simulink library "AEMS_Standard_Library"  (R2016b)
settings: Solver=ode45  StartTime=0.0  StopTime=10.0  RelTol=1e-3
undefined symbols (not defined in the file or in its folder): BkPY, carto, Cbx_extegr, Cbx_lpegrsys, Cbx_portegr, Cnx_bnk_nr_conf, Cnx_cyl_nr_conf, ConfigManagement, configuration_management, Cxx_dcm_io_tmr_end_xxxx, Cxx_dcm_rt_tmr_end, Cxx_DID_xxxx_IO_max, Cxx_DID_xxxx_IO_min, Cxx_egrhsofs, Cxx_vmaniegi, DEM_DEBOUNCE_FREEZE, DEM_DTR_CTL_INVISIBLE, DEM_DTR_CTL_NORMAL, Dem_DtrId2_XXX, Dem_DtrId3_XXX, Dem_DtrId4_XXX, Dem_DtrId5_XXX, Dem_DtrId6_XXX, Dem_DtrId7_XXX, Dem_DtrId8_XXX, Dem_DtrId9_XXX, Dem_DtrId_XXX, Dem_EnableConditionId2_XXX, Dem_EnableConditionId3_XXX, Dem_EnableConditionId4_XXX, Dem_EnableConditionId5_XXX, Dem_EnableConditionId6_XXX, Dem_EnableConditionId7_XXX, Dem_EnableConditionId8_XXX, Dem_EnableConditionId_XXX, Dem_EventId, Dem_EventId2_XXX, Dem_EventId3_XXX, Dem_EventId4_XXX, Dem_EventId5_XXX, Dem_EventId6_XXX, Dem_EventId7_XXX, Dem_EventId8_XXX, Dem_EventId9_XXX, Dem_EventId_Device_Faulttype, Dem_EventId_XXX, DEM_IUMPR_GENERAL_DENOMINATOR, DEM_OPCYC_IGNITION, Dem_RatioId2_XXX, Dem_RatioId3_XXX, Dem_RatioId4_XXX, Dem_RatioId5_XXX, Dem_RatioId6_XXX, Dem_RatioId7_XXX, Dem_RatioId8_XXX, Dem_RatioId_XXX, Dem_StorageConditionId2_XXX, Dem_StorageConditionId3_XXX, Dem_StorageConditionId4_XXX, Dem_StorageConditionId5_XXX ... (+65)
libraries: AEMS_Standard_Library x477, simulink x2
(part 17 of 39)

== system AEMS_Standard_Library/FILTER/AEMS_FILTER_WITH_DELAY_CONTROL ==
  filter_param : Inport
  kp : Inport  Port=2
  input : Inport  Port=3
  timestep : Inport  Port=4
  AEMS_SLEW_RATE : AEMS_Standard_Library/DISCONTINUITIES/AEMS_SLEW_RATE  Tag=[LIB]
      settings: AttributesFormatString=%<MaskType>
  Constant1 : Constant  Value=true
  DivisionByZero : Subsystem  Tag=[LIB]
  First_Order_Filter : Subsystem
  First_Order_Filter1 : Subsystem
  First_Order_Filter2 : Subsystem
  LogicalOperator2 : Logic  Operator=NOT  Inputs=1  OutDataTypeStr=boolean
  MinMax1 : MinMax  Function=max  Inputs=2  OutDataTypeStr=Inherit: Inherit via back propagation  RndMeth=Zero  InputSameDT=on
  MinMax2 : MinMax  Inputs=2  OutDataTypeStr=Inherit: Inherit via back propagation  RndMeth=Zero  InputSameDT=on
  Product : Product  OutDataTypeStr=Inherit: Inherit via back propagation  RndMeth=Zero
  Sum : Sum  Inputs=+-  OutDataTypeStr=Inherit: Inherit via back propagation  RndMeth=Zero  InputSameDT=on
  Sum2 : Sum  OutDataTypeStr=Inherit: Inherit via back propagation  RndMeth=Zero  InputSameDT=on
  Sum3 : Sum  Inputs=-+  OutDataTypeStr=Inherit: Inherit via back propagation  RndMeth=Zero  InputSameDT=on
  Sum5 : Sum  OutDataTypeStr=Inherit: Inherit via back propagation  RndMeth=Zero  InputSameDT=on
  UnitDelay : UnitDelay  SampleTime=-1
      settings: AttributesFormatString=IC = %<X0>
  UnitDelay1 : UnitDelay  SampleTime=-1
      settings: AttributesFormatString=IC = %<X0>
  Unit_Delay1 : UnitDelay  InitialCondition=false  SampleTime=-1
      settings: AttributesFormatString=IC = %<X0>
  g2 : Constant  Value=0  OutDataTypeStr=Inherit: Inherit via back propagation
  g4 : Constant  Value=0  OutDataTypeStr=Inherit: Inherit via back propagation
  g6 : Constant  Value=0  OutDataTypeStr=Inherit: Inherit via back propagation
  output : Outport
  wires:
  First_Order_Filter1/1(output) -> First_Order_Filter2/2(input)
  First_Order_Filter/1(output) -> First_Order_Filter1/2(input)
  filter_param/1 -> First_Order_Filter/1(filter_parameter), First_Order_Filter1/1(filter_parameter), First_Order_Filter2/1(filter_parameter)
  LogicalOperator2/1 -> First_Order_Filter/3(initial), First_Order_Filter1/3(initial), First_Order_Filter2/3(initial)
  Unit_Delay1/1 -> LogicalOperator2/1
  Constant1/1 -> Unit_Delay1/1
  First_Order_Filter2/1(output) -> UnitDelay1/1, Sum3/2
  input/1 -> AEMS_SLEW_RATE/2, Sum/1, First_Order_Filter/2(input)
  Sum3/1 -> DivisionByZero/2(num)
  Sum5/1 -> MinMax1/1
  DivisionByZero/1(ans) -> Sum5/1, Sum2/1
  UnitDelay/1 -> Sum/2
  MinMax1/1 -> AEMS_SLEW_RATE/1
  MinMax2/1 -> AEMS_SLEW_RATE/3
  kp/1 -> Product/2
  Sum/1 -> Product/1
  UnitDelay1/1 -> Sum3/1
  g2/1 -> MinMax1/2
  g4/1 -> MinMax2/2
  AEMS_SLEW_RATE/1 -> output/1, UnitDelay/1
  timestep/1 -> AEMS_SLEW_RATE/4, DivisionByZero/3(den)
  Sum2/1 -> MinMax2/1
  Product/1 -> Sum5/2, Sum2/2
  g6/1 -> DivisionByZero/1(ans_of_0div)

== system AEMS_Standard_Library/FILTER/AEMS_FIRST_ORDER_FILTER_RST ==
  Filter_param : Inport
  Input : Inport  Port=2
  IC : Inport  Port=3
  R : Inport  Port=4
  AEMS_UNITDELAY_RESET_EXTERNALIC : AEMS_Standard_Library/DISCRETE/AEMS_UNITDELAY_RESET_EXTERNALIC  Tag=[LIB]
      settings: AttributesFormatString=%<MaskType>
  Constant1 : Constant  Value=true
  Constant2 : Constant  OutDataTypeStr=Inherit: Inherit via back propagation
  LogicalOperator1 : Logic  Operator=OR  OutDataTypeStr=boolean
  LogicalOperator2 : Logic  Operator=NOT  Inputs=1  OutDataTypeStr=boolean
  Product1 : Product  OutDataTypeStr=single  RndMeth=Zero
  Product2 : Product  OutDataTypeStr=single  RndMeth=Zero
  Sum : Sum  Inputs=+-  OutDataTypeStr=single  RndMeth=Zero  InputSameDT=on
  Sum1 : Sum  OutDataTypeStr=single  RndMeth=Zero  InputSameDT=on
  Switch : Switch  Criteria=u2 ~= 0  RndMeth=Zero  SaturateOnIntegerOverflow=on  InputSameDT=on
      settings: AttributesFormatString=Criteria=%<Criteria>
  Unit_Delay1 : UnitDelay  InitialCondition=false  SampleTime=-1
      settings: AttributesFormatString=<initial=%<InitialCondition>>
  Output : Outport
  wires:
  LogicalOperator2/1 -> LogicalOperator1/2
  LogicalOperator1/1 -> Switch/2
  R/1 -> AEMS_UNITDELAY_RESET_EXTERNALIC/2, LogicalOperator1/1
  Switch/1 -> AEMS_UNITDELAY_RESET_EXTERNALIC/1, Output/1
  IC/1 -> AEMS_UNITDELAY_RESET_EXTERNALIC/3, Switch/1
  Sum1/1 -> Switch/3
  Product2/1 -> Sum1/2
  Product1/1 -> Sum1/1
  Unit_Delay1/1 -> LogicalOperator2/1
  Constant1/1 -> Unit_Delay1/1
  Filter_param/1 -> Product2/1, Sum/2
  Constant2/1 -> Sum/1
  Input/1 -> Product2/2
  Sum/1 -> Product1/2
  AEMS_UNITDELAY_RESET_EXTERNALIC/1 -> Product1/1

== system AEMS_Standard_Library/FILTER/AEMS_FORWARD_EULER_INTEGRATOR_WITH_RESET ==
  note: External reset: "level"
  note: Forward Euler: y(n) = x(n-1)*T*K + y(n-1)
  x : Inport
  Reset : Inport  Port=2
  IC : Inport  Port=3
  uppersaturation : Inport  Port=4
  lowersaturation : Inport  Port=5
  Sample_Time : Inport  Port=6
  Gain_K : Inport  Port=7
  AEMS_CLAMP1 : AEMS_Standard_Library/MATH/AEMS_CLAMP  Tag=[LIB]
      settings: AttributesFormatString=%<MaskType>
  AEMS_UNITDELAY_EXTERNALIC : AEMS_Standard_Library/DISCRETE/AEMS_UNITDELAY_EXTERNALIC  Tag=[LIB]
      settings: AttributesFormatString=%<MaskType>
  Add1 : Sum  OutDataTypeStr=Inherit: Inherit via back propagation  RndMeth=Zero  InputSameDT=on
  LogicalOperator1 : Logic  Operator=OR  OutDataTypeStr=boolean
  Product1 : Product  OutDataTypeStr=Inherit: Inherit via back propagation  RndMeth=Zero
  Product2 : Product  OutDataTypeStr=Inherit: Inherit via back propagation  RndMeth=Zero
  Switch1 : Switch  Criteria=u2 ~= 0  RndMeth=Zero  InputSameDT=on
      settings: AttributesFormatString=Criteria=%<Criteria>
  UnitDelay1 : UnitDelay  SampleTime=-1
      settings: AttributesFormatString=IC = %<X0>
  UnitDelay2 : UnitDelay  SampleTime=-1
      settings: AttributesFormatString=IC = %<X0>
  y : Outport
  wires:
  AEMS_UNITDELAY_EXTERNALIC/1 -> Add1/1
  Product2/1 -> Add1/2
  lowersaturation/1 -> AEMS_CLAMP1/3
  uppersaturation/1 -> AEMS_CLAMP1/1
  Reset/1 -> LogicalOperator1/1, UnitDelay1/1
  UnitDelay1/1 -> LogicalOperator1/2
  IC/1 -> Switch1/1, AEMS_UNITDELAY_EXTERNALIC/2
  x/1 -> UnitDelay2/1
  Sample_Time/1 -> Product1/2
  UnitDelay2/1 -> Product1/1
  Product1/1 -> Product2/1
  Gain_K/1 -> Product2/2
  Add1/1 -> Switch1/3
  LogicalOperator1/1 -> Switch1/2
  Switch1/1 -> AEMS_CLAMP1/2
  AEMS_CLAMP1/1 -> AEMS_UNITDELAY_EXTERNALIC/1, y/1

== system AEMS_Standard_Library/FILTER/AEMS_TAU_TO_FILTER_PARAM ==
  note: Nxb_fil_para = [0.0 0.125 0.25 0.375 0.5 0.625 0.75 0.875 1.0]
  note: Nxp_fil_para = [1.0 0.882497 0.7788 0.687289 0.606531 0.535261 0.472366 0.416862 0.367879]
  Tau : Inport
  Timestep : Inport  Port=2
  AEMS_LUT_1D : AEMS_Standard_Library/LOOKUP_TABLES/AEMS_LUT_1D  Tag=[LIB]  map_x=Nxb_fil_para  map_z=Nxp_fil_para
      settings: AttributesFormatString=%<MaskType>\nBkPX=%<map_x>\nLUT=%<map_z>
  Constant1 : Constant  Value=0  OutDataTypeStr=single
  Constant13 : Constant  OutDataTypeStr=single
  Constant2 : Constant  Value=1.1920929e-07  OutDataTypeStr=single
  Constant3 : Constant  OutDataTypeStr=single
  Divide : Product  Inputs=*/  OutDataTypeStr=Inherit: Inherit via back propagation  RndMeth=Zero
  MinMax : MinMax  Function=max  Inputs=2  OutDataTypeStr=Inherit: Inherit via back propagation  RndMeth=Zero  InputSameDT=on
  RelationalOperator : RelationalOperator  Operator=>  OutDataTypeStr=boolean  RndMeth=Nearest  InputSameDT=on
  Saturation : Saturate  UpperLimit=1  LowerLimit=0  RndMeth=Zero
      settings: AttributesFormatString=L_Limit = %<LowerLimit>\nU_Limit = %<UpperLimit>
  Sum1 : Sum  Inputs=+-  OutDataTypeStr=Inherit: Inherit via back propagation  RndMeth=Zero  InputSameDT=on
  Switch : Switch  Criteria=u2 ~= 0  RndMeth=Zero  SaturateOnIntegerOverflow=on  InputSameDT=on
      settings: AttributesFormatString=Criteria=%<Criteria>
  Filter_param : Outport
  wires:
  Sum1/1 -> Switch/1
  RelationalOperator/1 -> Switch/2
  Constant1/1 -> RelationalOperator/2
  Divide/1 -> Saturation/1
  Tau/1 -> MinMax/1, RelationalOperator/1
  Timestep/1 -> Divide/1
  Constant2/1 -> MinMax/2
  MinMax/1 -> Divide/2
  Saturation/1 -> AEMS_LUT_1D/1
  Switch/1 -> Filter_param/1
  Constant13/1 -> Sum1/1
  AEMS_LUT_1D/1 -> Sum1/2
  Constant3/1 -> Switch/3

== system AEMS_Standard_Library/FILTER/AEMS_TAU_TO_FILTER_PARAM_EXP ==
  Tau : Inport
  Timestep : Inport  Port=2
  Constant : Constant  Value=-1  OutDataTypeStr=Inherit: Inherit via back propagation
  Constant1 : Constant  Value=0  OutDataTypeStr=single
  Constant13 : Constant  OutDataTypeStr=single
  Constant2 : Constant  Value=1.1920929e-07  OutDataTypeStr=single
  Constant3 : Constant  OutDataTypeStr=single
  Divide : Product  Inputs=*/  OutDataTypeStr=Inherit: Inherit via back propagation  RndMeth=Zero
  MathFunction : Math  RndMeth=Zero  SaturateOnIntegerOverflow=on
  MinMax : MinMax  Function=max  Inputs=2  OutDataTypeStr=Inherit: Inherit via back propagation  RndMeth=Zero  InputSameDT=on
  Product : Product  OutDataTypeStr=Inherit: Inherit via back propagation  RndMeth=Zero
  RelationalOperator : RelationalOperator  Operator=>  OutDataTypeStr=boolean  RndMeth=Nearest  InputSameDT=on
  Saturation : Saturate  UpperLimit=1  LowerLimit=0  RndMeth=Zero
      settings: AttributesFormatString=L_Limit = %<LowerLimit>\nU_Limit = %<UpperLimit>
  Sum1 : Sum  Inputs=+-  OutDataTypeStr=Inherit: Inherit via back propagation  RndMeth=Zero  InputSameDT=on
  Switch : Switch  Criteria=u2 ~= 0  RndMeth=Zero  SaturateOnIntegerOverflow=on  InputSameDT=on
      settings: AttributesFormatString=Criteria=%<Criteria>
  Filter_param : Outport
  wires:
  Sum1/1 -> Switch/1
  RelationalOperator/1 -> Switch/2
  Constant1/1 -> RelationalOperator/2
  Divide/1 -> Saturation/1
  Tau/1 -> MinMax/1, RelationalOperator/1
  Timestep/1 -> Divide/1
  Constant2/1 -> MinMax/2
  MinMax/1 -> Divide/2
  Product/1 -> MathFunction/1
  Switch/1 -> Filter_param/1
  Constant13/1 -> Sum1/1
  MathFunction/1 -> Sum1/2
  Constant3/1 -> Switch/3
  Saturation/1 -> Product/1
  Constant/1 -> Product/2

== system AEMS_Standard_Library/FLAG/AEMS_SRFLIPFLOP ==
  S : Inport
  R : Inport  Port=2
  LogicalOperator : Logic  Operator=NOR  OutDataTypeStr=boolean
  LogicalOperator1 : Logic  Operator=NOR  OutDataTypeStr=boolean
  UnitDelay1 : UnitDelay  InitialCondition=InitValue  SampleTime=-1
      settings: AttributesFormatString=IC = %<X0>
  Q : Outport  InitialOutput=1
  wires:
  UnitDelay1/1 -> LogicalOperator/1
  S/1 -> LogicalOperator/2
  LogicalOperator/1 -> LogicalOperator1/1
  LogicalOperator1/1 -> Q/1, UnitDelay1/1
  R/1 -> LogicalOperator1/2

== system AEMS_Standard_Library/HYSTERESIS/AEMS_HYST_DELTARIGHT ==
  note: Hysteresis Model
  val : Inport
      settings: AttributesFormatString=<tsample=%<SampleTime>>
  thrs : Inport  Port=2
      settings: AttributesFormatString=<tsample=%<SampleTime>>
  hysw : Inport  Port=3
      settings: AttributesFormatString=<tsample=%<SampleTime>>
  NOT : Logic  Operator=NOT  Inputs=1  OutDataTypeStr=boolean
  Sum : Sum  SaturateOnIntegerOverflow=on
  Switch : Switch  Criteria=u2 ~= 0  SaturateOnIntegerOverflow=on  InputSameDT=on
      settings: AttributesFormatString=Criteria=%<Criteria>
  Unit Delay : UnitDelay  SampleTime=-1
      settings: AttributesFormatString=<initial=%<X0>>
  hflg=OFF : RelationalOperator  Operator=<=  OutDataTypeStr=boolean  RndMeth=Nearest  InputSameDT=on
  hflg=ON : RelationalOperator  Operator=>  OutDataTypeStr=boolean  RndMeth=Nearest  InputSameDT=on
  flg_ret : Outport
  wires:
  Unit Delay/1 -> Switch/2
  hflg=OFF/1 -> Switch/3
  hflg=ON/1 -> Switch/1
  hysw/1 -> Sum/2  "hysw"
  Switch/1 -> NOT/1
  NOT/1 -> Unit Delay/1, flg_ret/1  "flg_ret"
  Sum/1 -> hflg=ON/2
  thrs/1 -> hflg=ON/1, hflg=OFF/2  "thrs"
  val/1 -> Sum/1, hflg=OFF/1  "val"

== system AEMS_Standard_Library/HYSTERESIS/AEMS_HYST_LEFTDELTA ==
  note: Hysteresis Model
  val : Inport
      settings: AttributesFormatString=<tsample=%<SampleTime>>
  thrs : Inport  Port=2
      settings: AttributesFormatString=<tsample=%<SampleTime>>
  hysw : Inport  Port=3
      settings: AttributesFormatString=<tsample=%<SampleTime>>
  NOT : Logic  Operator=NOT  Inputs=1  OutDataTypeStr=boolean
  Sum : Sum  Inputs=+-  SaturateOnIntegerOverflow=on
  Switch : Switch  Criteria=u2 ~= 0  SaturateOnIntegerOverflow=on  InputSameDT=on
      settings: AttributesFormatString=Criteria=%<Criteria>
  Unit Delay : UnitDelay  SampleTime=-1
      settings: AttributesFormatString=<initial=%<X0>>
  hflg=OFF : RelationalOperator  Operator=<  OutDataTypeStr=boolean  RndMeth=Nearest  InputSameDT=on
  hflg=ON : RelationalOperator  OutDataTypeStr=boolean  RndMeth=Nearest  InputSameDT=on
  flg_ret : Outport
  wires:
  Unit Delay/1 -> NOT/1
  NOT/1 -> Switch/2
  hysw/1 -> Sum/2  "hysw"
  Sum/1 -> hflg=OFF/2
  hflg=OFF/1 -> Switch/1
  hflg=ON/1 -> Switch/3
  Switch/1 -> Unit Delay/1, flg_ret/1  "flg_ret"
  val/1 -> Sum/1, hflg=ON/1  "val"
  thrs/1 -> hflg=OFF/1, hflg=ON/2  "thrs"

== system AEMS_Standard_Library/HYSTERESIS/AEMS_HYST_LEFTRIGHT ==
  Input : Inport  Tag=AM,In,0,1,Name,C;CMP,Port,PortWidth,SampleTime;
  Low_Threshold : Inport  Tag=AM,In,0,1,Name,C;CMP,Port,PortWidth,SampleTime;  Port=2
  High_Threshold : Inport  Tag=AM,In,0,1,Name,C;CMP,Port,PortWidth,SampleTime;  Port=3
  Constant1 : Constant  Value=false
  Logical_Operator2 : Logic  Operator=OR  OutDataTypeStr=boolean
  Relational_Operator : RelationalOperator  Tag=AM,Std,2,1;CMP,Operator;  Operator=>  OutDataTypeStr=boolean  RndMeth=Nearest  InputSameDT=on
  Relational_Operator1 : RelationalOperator  Tag=AM,Std,2,1;CMP,Operator;  Operator=>  OutDataTypeStr=boolean  RndMeth=Nearest  InputSameDT=on
  Switch2 : Switch  Tag=GEN,Threshold;AM,Switch,2,1;CMP,Threshold;  Criteria=u2 ~= 0  RndMeth=Zero  SaturateOnIntegerOverflow=on  InputSameDT=on
      settings: AttributesFormatString=Criteria=%<Criteria>
  Unit Delay : UnitDelay  InitialCondition=InitValue  SampleTime=-1
      settings: AttributesFormatString=<initial=%<X0>>
  Output : Outport  Tag=AM,Out,1,0,Name,NC;CMP,Port,OutputWhenDisabled,InitialOutput;
  wires:
  Low_Threshold/1 -> Relational_Operator/1
  High_Threshold/1 -> Relational_Operator1/2
  Input/1 -> Relational_Operator/2, Relational_Operator1/1
  Relational_Operator/1 -> Switch2/2
  Relational_Operator1/1 -> Logical_Operator2/1
  Constant1/1 -> Switch2/1
  Switch2/1 -> Unit Delay/1, Output/1
  Logical_Operator2/1 -> Switch2/3
  Unit Delay/1 -> Logical_Operator2/2

== system AEMS_Standard_Library/LOOKUP_TABLES/AEMS_DIRECTLU_1D ==
  Index_Ratio : Inport
  Table : Inport  Port=2
  Bus Selector : BusSelector  OutputSignals=Index,Ratio
  Interp (1D) Using PreLookUp : Interpolation_n-D  NumberOfTableDimensions=1  TableSource=Input port  Table=LUT  ExtrapMethod=Clip  RemoveProtectionIndex=on  ValidIndexMayReachLast=on  OutDataTypeStr=Inherit: Inherit via back propagation  RndMeth=Zero  SaturateOnIntegerOverflow=on  TableDataTypeStr=Inherit: Inherit from 'Table data'
      settings: AttributesFormatString=Interpolation method : %<InterpMethod>\nExtrapolation method : %<ExtrapMethod>\nRounding mode : %<RndMeth>  InputPortMap=u0,u1,p2
  Value : Outport
  wires:
  Table/1 -> Interp (1D) Using PreLookUp/3
  Index_Ratio/1 -> Bus Selector/1
  Bus Selector/2 -> Interp (1D) Using PreLookUp/2  "<Ratio>"
  Bus Selector/1 -> Interp (1D) Using PreLookUp/1  "<Index>"
  Interp (1D) Using PreLookUp/1 -> Value/1

== system AEMS_Standard_Library/LOOKUP_TABLES/AEMS_DIRECTLU_2D ==
  Index_Ratio_X : Inport
  Index_Ratio_Y : Inport  Port=2
  MAP : Inport  Port=3
  Bus Selector X : BusSelector  OutputSignals=Index,Ratio
  Bus Selector Y : BusSelector  OutputSignals=Index,Ratio
  Interp (2D) Using PreLookUp : Interpolation_n-D  TableSource=Input port  Table=LUT  ExtrapMethod=Clip  RemoveProtectionIndex=on  ValidIndexMayReachLast=on  OutDataTypeStr=Inherit: Inherit via back propagation  RndMeth=Zero  SaturateOnIntegerOverflow=on  TableDataTypeStr=Inherit: Inherit from 'Table data'
      settings: AttributesFormatString=Interpolation method : %<InterpMethod>\nExtrapolation method : %<ExtrapMethod>\nRounding mode : %<RndMeth>  InputPortMap=u0,u1,u2,u3,p2
  Value : Outport
  wires:
  Index_Ratio_X/1 -> Bus Selector X/1
  Index_Ratio_Y/1 -> Bus Selector Y/1
  Interp (2D) Using PreLookUp/1 -> Value/1
  Bus Selector X/1 -> Interp (2D) Using PreLookUp/1  "<Index>"
  Bus Selector X/2 -> Interp (2D) Using PreLookUp/2  "<Ratio>"
  Bus Selector Y/1 -> Interp (2D) Using PreLookUp/3  "<Index>"
  Bus Selector Y/2 -> Interp (2D) Using PreLookUp/4  "<Ratio>"
  MAP/1 -> Interp (2D) Using PreLookUp/5

== system AEMS_Standard_Library/LOOKUP_TABLES/AEMS_DIRECTLU_INDEXED_1D ==
  Index_Ratio : Inport
  Table : Inport  Port=2
  Bus Selector : BusSelector  OutputSignals=Index
  Direct Look-Up Table (1D) : LookupNDDirect  NumberOfTableDimensions=1  TableIsInput=on  Table=LUT  DiagnosticForOutOfRangeInput=None
      settings: LockScale=on
  Value : Outport
  wires:
  Direct Look-Up Table (1D)/1 -> Value/1
  Bus Selector/1 -> Direct Look-Up Table (1D)/1  "<Index>"
  Index_Ratio/1 -> Bus Selector/1
  Table/1 -> Direct Look-Up Table (1D)/2

== system AEMS_Standard_Library/LOOKUP_TABLES/AEMS_DIRECTLU_INDEXED_2D ==
  Index_Ratio_X : Inport
  Index_Ratio_Y : Inport  Port=2
  MAP : Inport  Port=3
  Bus Selector X : BusSelector  OutputSignals=Index
  Bus Selector Y : BusSelector  OutputSignals=Index
  Direct Look-Up Table (2D) : LookupNDDirect  TableIsInput=on  Table=LUT  DiagnosticForOutOfRangeInput=None
      settings: LockScale=on
  Value : Outport
  wires:
  Index_Ratio_X/1 -> Bus Selector X/1
  Index_Ratio_Y/1 -> Bus Selector Y/1
  Direct Look-Up Table (2D)/1 -> Value/1
  Bus Selector X/1 -> Direct Look-Up Table (2D)/1  "<Index>"
  Bus Selector Y/1 -> Direct Look-Up Table (2D)/2  "<Index>"
  MAP/1 -> Direct Look-Up Table (2D)/3

== system AEMS_Standard_Library/LOOKUP_TABLES/AEMS_DYNAMIC_LUT_1D ==
  Var : Inport
  BkPX : Inport  Port=2
  LUT : Inport  Port=3
  LookupTableDynamic : simulink/Lookup Tables/Lookup Table Dynamic  LookUpMeth=Interpolation-Use End Values  OutDataType=fixdt('double')  OutScaling=[]  OutDataTypeStr=Inherit: Inherit via back propagation  DoSatur=off
      settings: AttributesFormatString=LU Method : %<LookUpMeth>\nRounding mode : %<RndMeth>
  Interp1D : Outport
  wires:
  LookupTableDynamic/1 -> Interp1D/1
  Var/1 -> LookupTableDynamic/1
  BkPX/1 -> LookupTableDynamic/2
  LUT/1 -> LookupTableDynamic/3

== system AEMS_Standard_Library/LOOKUP_TABLES/AEMS_INDEXED_LUT_1D ==
  Var : Inport
  LookupTableIndexed1D : Lookup_n-D  NumberOfTableDimensions=1  BreakpointsForDimension1=map_x  BreakpointsForDimension2=BkPY  BreakpointsForDimension1DataTypeStr=Inherit: Inherit from 'Breakpoint data'  BreakpointsForDimension2DataTypeStr=Inherit: Inherit from 'Breakpoint data'  Table=map_z  TableDataTypeStr=Inherit: Inherit from 'Table data'  InterpMethod=Flat  ExtrapMethod=Clip  UseLastTableValue=on  OutDataTypeStr=Inherit: Inherit via back propagation  RndMeth=Zero  SaturateOnIntegerOverflow=on
      settings: AttributesFormatString="Interpolation method : %<interpMethod>\\nExtrapolation method : %<extrapMethod>\\nBkPX = %<bp1>\\nMAP  = %<tableData>"
  Index1D : Outport
  wires:
  Var/1 -> LookupTableIndexed1D/1
  LookupTableIndexed1D/1 -> Index1D/1

== system AEMS_Standard_Library/LOOKUP_TABLES/AEMS_INDEXED_LUT_1D_TOL ==
  Var : Inport
  AEMS_SRFLIPFLOP : AEMS_Standard_Library/FLAG/AEMS_SRFLIPFLOP  Tag=[LIB]  init=true
      settings: AttributesFormatString=|
      | %<MaskType>
      | Initial condition (state of Q): %<init>
  Constant6 : Constant
  Logical Operator1 : Logic  OutDataTypeStr=boolean
  Lookup Table Indexed (1D) : Lookup_n-D  NumberOfTableDimensions=1  BreakpointsForDimension1=map_x  BreakpointsForDimension2=BkPY  BreakpointsForDimension1DataTypeStr=Inherit: Inherit from 'Breakpoint data'  BreakpointsForDimension2DataTypeStr=Inherit: Inherit from 'Breakpoint data'  Table=map_z  TableDataTypeStr=Inherit: Inherit from 'Table data'  InterpMethod=Flat  ExtrapMethod=Clip  UseLastTableValue=on  OutDataTypeStr=Inherit: Inherit via back propagation  RndMeth=Zero  SaturateOnIntegerOverflow=on
      settings: AttributesFormatString="Interpolation method : %<interpMethod>\\nExtrapolation method : %<extrapMethod>\\nBkPX = %<bp1>\\nMAP  = %<tableData>"
  PreLookUpX : Subsystem
  PreLookUpX+Tol : Subsystem
  Relational Operator1 : RelationalOperator  Operator=~=  OutDataTypeStr=boolean  RndMeth=Nearest  InputSameDT=on
  Relational Operator3 : RelationalOperator  Operator===  OutDataTypeStr=boolean  RndMeth=Nearest  InputSameDT=on
  Relational Operator5 : RelationalOperator  Operator===  OutDataTypeStr=boolean  RndMeth=Nearest  InputSameDT=on
  Sum2 : Sum  SaturateOnIntegerOverflow=on
  Sum6 : Sum  Inputs=+-  RndMeth=Zero  SaturateOnIntegerOverflow=on
  Switch : Switch  Criteria=u2 ~= 0  SaturateOnIntegerOverflow=on
      settings: AttributesFormatString=Criteria=%<Criteria>
  Unit Delay1 : UnitDelay  SampleTime=-1
  Unit Delay2 : UnitDelay  SampleTime=-1
  X_Tolerance : Constant  Value=Tolerance
  Result : Outport
  wires:
  X_Tolerance/1 -> Sum2/1
  PreLookUpX+Tol/1(k) -> Relational Operator3/1
  Lookup Table Indexed (1D)/1 -> Result/1
  Switch/1 -> Lookup Table Indexed (1D)/1
  Relational Operator3/1 -> Unit Delay2/1, Relational Operator1/1, AEMS_SRFLIPFLOP/2
  AEMS_SRFLIPFLOP/1 -> Switch/2
  Unit Delay2/1 -> Relational Operator1/2
  Relational Operator1/1 -> Logical Operator1/2
  Relational Operator5/1 -> Logical Operator1/1
  Logical Operator1/1 -> AEMS_SRFLIPFLOP/1
  Var/1 -> PreLookUpX/1(u), Switch/3, Sum2/2
  Sum2/1 -> PreLookUpX+Tol/1(u), Switch/1
  Sum6/1 -> Relational Operator5/1
  Constant6/1 -> Relational Operator5/2
  Unit Delay1/1 -> Sum6/1
  PreLookUpX/1(k) -> Sum6/2, Unit Delay1/1, Relational Operator3/2

== system AEMS_Standard_Library/LOOKUP_TABLES/AEMS_INDEXED_LUT_2D ==
  VarX : Inport
  VarY : Inport  Port=2
  Lookup Table Indexed (2D) : Lookup_n-D  BreakpointsForDimension1=map_x  BreakpointsForDimension2=map_y  BreakpointsForDimension1DataTypeStr=Inherit: Inherit from 'Breakpoint data'  BreakpointsForDimension2DataTypeStr=Inherit: Inherit from 'Breakpoint data'  Table=carto  TableDataTypeStr=Inherit: Inherit from 'Table data'  InterpMethod=Flat  ExtrapMethod=Clip  UseLastTableValue=on  OutDataTypeStr=Inherit: Inherit via back propagation  RndMeth=Zero  SaturateOnIntegerOverflow=on
      settings: AttributesFormatString="Interpolation method : %<interpMethod>\\nExtrapolation Method : %<extrapMethod>\\nBkPX = %<bp1>\\nBkPY =  %<bp2>\\nMAP  = %<tableData>"
  Index2D : Outport
  wires:
  Lookup Table Indexed (2D)/1 -> Index2D/1
  VarX/1 -> Lookup Table Indexed (2D)/1
  VarY/1 -> Lookup Table Indexed (2D)/2

== system AEMS_Standard_Library/LOOKUP_TABLES/AEMS_INDEXED_LUT_2D_TOL ==
  VarX : Inport
  VarY : Inport  Port=2
  AEMS_SRFLIPFLOPIC : AEMS_Standard_Library/FLAG/AEMS_SRFLIPFLOP  Tag=[LIB]  init=true
      settings: AttributesFormatString=|
      | %<MaskType>
      | Initial condition (state of Q): %<init>
  AEMS_SRFLIPFLOPIC1 : AEMS_Standard_Library/FLAG/AEMS_SRFLIPFLOP  Tag=[LIB]  init=true
      settings: AttributesFormatString=|
      | %<MaskType>
      | Initial condition (state of Q): %<init>
  Constant1 : Constant
  Constant6 : Constant
  Logical Operator1 : Logic  AllPortsSameDT=off
  Logical Operator2 : Logic  AllPortsSameDT=off
  Lookup Table Indexed (2D) : Lookup_n-D  BreakpointsForDimension1=map_x  BreakpointsForDimension2=map_y  BreakpointsForDimension1DataTypeStr=Inherit: Inherit from 'Breakpoint data'  BreakpointsForDimension2DataTypeStr=Inherit: Inherit from 'Breakpoint data'  Table=carto  TableDataTypeStr=Inherit: Inherit from 'Table data'  InterpMethod=Flat  ExtrapMethod=Clip  UseLastTableValue=on  OutDataTypeStr=Inherit: Inherit via back propagation  RndMeth=Zero  SaturateOnIntegerOverflow=on
      settings: AttributesFormatString="Interpolation method : %<interpMethod>\\nExtrapolation Method : %<extrapMethod>\\nBkPX = %<bp1>\\nBkPY =  %<bp2>\\nMAP  = %<tableData>"
  PreLookUpX : Subsystem
  PreLookUpX+Tol : Subsystem
  PreLookUpY : Subsystem
  PreLookUpY+Tol1 : Subsystem
  Relational Operator1 : RelationalOperator  Operator=~=  OutDataTypeStr=boolean  RndMeth=Nearest
  Relational Operator2 : RelationalOperator  Operator=~=  OutDataTypeStr=boolean  RndMeth=Nearest
  Relational Operator{3..6} (4 alike) : RelationalOperator  Operator===  OutDataTypeStr=boolean  RndMeth=Nearest
  Sum1 : Sum  SaturateOnIntegerOverflow=on
  Sum2 : Sum  SaturateOnIntegerOverflow=on
  Sum3 : Sum  Inputs=+-  RndMeth=Zero  SaturateOnIntegerOverflow=on
  Sum6 : Sum  Inputs=+-  RndMeth=Zero  SaturateOnIntegerOverflow=on
  Switch1 : Switch  Threshold=0.5  SaturateOnIntegerOverflow=on
      settings: AttributesFormatString=<threshold=%<threshold>>\n
  Switch2 : Switch  Threshold=0.5  SaturateOnIntegerOverflow=on
      settings: AttributesFormatString=<threshold=%<threshold>>\n
  Unit Delay{1..4} (4 alike) : UnitDelay  SampleTime=-1
  X_Tolerance : Constant  Tag=AM,Constant,0,1,Value;CMP,Value;  Value=X_Tolerance
  Y_Tolerance2 : Constant  Tag=AM,Constant,0,1,Value;CMP,Value;  Value=Y_Tolerance
  Result : Outport
  wires:
  Y_Tolerance2/1 -> Sum1/1
  PreLookUpY+Tol1/1(k) -> Relational Operator4/1
  Relational Operator4/1 -> AEMS_SRFLIPFLOPIC1/2, Unit Delay4/1, Relational Operator2/1
  AEMS_SRFLIPFLOPIC1/1 -> Switch1/2
  Unit Delay4/1 -> Relational Operator2/2
  Relational Operator2/1 -> Logical Operator2/2
  Relational Operator6/1 -> Logical Operator2/1
  Logical Operator2/1 -> AEMS_SRFLIPFLOPIC1/1
  VarY/1 -> Switch1/3, Sum1/2, PreLookUpY/1(u)
  Sum1/1 -> Switch1/1, PreLookUpY+Tol1/1(u)
  Sum3/1 -> Relational Operator6/1
  Constant1/1 -> Relational Operator6/2
  Unit Delay3/1 -> Sum3/1
  PreLookUpY/1(k) -> Sum3/2, Unit Delay3/1, Relational Operator4/2
  X_Tolerance/1 -> Sum2/1
  PreLookUpX+Tol/1(k) -> Relational Operator3/1
  Lookup Table Indexed (2D)/1 -> Result/1
  Switch1/1 -> Lookup Table Indexed (2D)/2
  Switch2/1 -> Lookup Table Indexed (2D)/1
  Relational Operator3/1 -> AEMS_SRFLIPFLOPIC/2, Unit Delay2/1, Relational Operator1/1
  AEMS_SRFLIPFLOPIC/1 -> Switch2/2
  Unit Delay2/1 -> Relational Operator1/2
  Relational Operator1/1 -> Logical Operator1/2
  Relational Operator5/1 -> Logical Operator1/1
  Logical Operator1/1 -> AEMS_SRFLIPFLOPIC/1
  VarX/1 -> PreLookUpX/1(u), Switch2/3, Sum2/2
  Sum2/1 -> PreLookUpX+Tol/1(u), Switch2/1
  Sum6/1 -> Relational Operator5/1
  Constant6/1 -> Relational Operator5/2
  Unit Delay1/1 -> Sum6/1
  PreLookUpX/1(k) -> Sum6/2, Unit Delay1/1, Relational Operator3/2

== system AEMS_Standard_Library/LOOKUP_TABLES/AEMS_INTERP ==
  input_of_ratio_1 : Inport
      settings: AttributesFormatString=<tsample=%<sampleTime>>
  interpolate_ratio : Inport  Port=2
      settings: AttributesFormatString=<tsample=%<sampleTime>>
  input_of_ratio_0 : Inport  Port=3
      settings: AttributesFormatString=<tsample=%<sampleTime>>
  Constant1 : Constant  OutDataTypeStr=Inherit: Inherit via back propagation
  Product : Product  SaturateOnIntegerOverflow=on  RndMeth=Zero  InputSameDT=on
  Product1 : Product  SaturateOnIntegerOverflow=on  RndMeth=Zero  InputSameDT=on
  Saturation : Saturate  UpperLimit=1  LowerLimit=0
      settings: AttributesFormatString=<limits=%<UpperLimit>/%<LowerLimit>>
  Sum : Sum  Inputs=-+  SaturateOnIntegerOverflow=on  InputSameDT=on
  Sum1 : Sum  SaturateOnIntegerOverflow=on  InputSameDT=on
  output : Outport
  wires:
  Sum1/1 -> output/1  "output"
  Constant1/1 -> Sum/2
  input_of_ratio_0/1 -> Product1/2  "input_of_ratio_0"
  Product1/1 -> Sum1/2
  Product/1 -> Sum1/1
  Sum/1 -> Product1/1
  interpolate_ratio/1 -> Saturation/1  "interpolate_ratio"
  input_of_ratio_1/1 -> Product/1  "input_of_ratio_1"
  Saturation/1 -> Product/2, Sum/1  "limited_interpolate_ratio"

== system AEMS_Standard_Library/LOOKUP_TABLES/AEMS_ITP3D ==
  Vxx_fac : Inport
  Vxx_in1 : Inport  Port=2
  Vxx_in2 : Inport  Port=3
  Vxx_in3 : Inport  Port=4
  DataTypeConversion : DataTypeConversion  OutDataTypeStr=uint8  SaturateOnIntegerOverflow=on  RndMeth=Zero
  DataTypeConversion2 : DataTypeConversion  OutDataTypeStr=uint8  SaturateOnIntegerOverflow=on  RndMeth=Zero
  MultiportSwitch : MultiPortSwitch  RndMeth=Zero  SaturateOnIntegerOverflow=on  InputSameDT=on
      settings: AttributesFormatString=PortOrder=%<DataPortOrder>
  MultiportSwitch1 : MultiPortSwitch  RndMeth=Zero  SaturateOnIntegerOverflow=on  InputSameDT=on
      settings: AttributesFormatString=PortOrder=%<DataPortOrder>
  Product : Product  OutDataTypeStr=Inherit: Inherit via back propagation  RndMeth=Zero
  RoundingFunction : Rounding
      settings: AttributesFormatString=Function = %<Operator>
  RoundingFunction1 : Rounding  Operator=ceil
      settings: AttributesFormatString=Function = %<Operator>
  Saturation : Saturate  UpperLimit=3  LowerLimit=1  RndMeth=Zero
      settings: AttributesFormatString=L_Limit = %<LowerLimit>\nU_Limit = %<UpperLimit>
  Sum : Sum  Inputs=+-  OutDataTypeStr=Inherit: Inherit via back propagation  RndMeth=Zero  InputSameDT=on
  Sum1 : Sum  Inputs=+-  OutDataTypeStr=Inherit: Inherit via back propagation  RndMeth=Zero  InputSameDT=on
  Sum2 : Sum  OutDataTypeStr=Inherit: Inherit via back propagation  RndMeth=Zero  InputSameDT=on
  Vxx_out : Outport
  wires:
  DataTypeConversion2/1 -> MultiportSwitch/1
  DataTypeConversion/1 -> MultiportSwitch1/1
  MultiportSwitch/1 -> Sum2/2, Sum1/2
  RoundingFunction/1 -> DataTypeConversion2/1, Sum/2
  RoundingFunction1/1 -> DataTypeConversion/1
  Vxx_in2/1 -> MultiportSwitch1/3, MultiportSwitch/3
  Vxx_in3/1 -> MultiportSwitch1/4, MultiportSwitch/4
  Sum1/1 -> Product/2
  MultiportSwitch1/1 -> Sum1/1
  Vxx_in1/1 -> MultiportSwitch1/2, MultiportSwitch/2
  Sum2/1 -> Vxx_out/1
  Product/1 -> Sum2/1
  Sum/1 -> Product/1
  Saturation/1 -> Sum/1, RoundingFunction/1, RoundingFunction1/1
  Vxx_fac/1 -> Saturation/1

== system AEMS_Standard_Library/LOOKUP_TABLES/AEMS_LUT_1D ==
  Var : Inport
  LookupTable1D : Lookup_n-D  NumberOfTableDimensions=1  BreakpointsForDimension1=map_x  BreakpointsForDimension2=BkPY  BreakpointsForDimension1DataTypeStr=Inherit: Inherit from 'Breakpoint data'  BreakpointsForDimension2DataTypeStr=Inherit: Inherit from 'Breakpoint data'  Table=map_z  TableDataTypeStr=Inherit: Inherit from 'Table data'  ExtrapMethod=Clip  UseLastTableValue=on  OutDataTypeStr=Inherit: Inherit via back propagation  RndMeth=Zero  SaturateOnIntegerOverflow=on
      settings: AttributesFormatString="Interpolation method : %<interpMethod>\\nExtrapolation method : %<extrapMethod>\\nBkPX = %<bp1>\\nMAP  = %<tableData>"
  Interp1D : Outport
  wires:
  Var/1 -> LookupTable1D/1
  LookupTable1D/1 -> Interp1D/1

== system AEMS_Standard_Library/LOOKUP_TABLES/AEMS_LUT_2D ==
  VarX : Inport
  VarY : Inport  Port=2
  Lookup Table (2D) : Lookup_n-D  BreakpointsForDimension1=map_x  BreakpointsForDimension2=map_y  BreakpointsForDimension1DataTypeStr=Inherit: Inherit from 'Breakpoint data'  BreakpointsForDimension2DataTypeStr=Inherit: Inherit from 'Breakpoint data'  Table=carto  TableDataTypeStr=Inherit: Inherit from 'Table data'  ExtrapMethod=Clip  UseLastTableValue=on  OutDataTypeStr=Inherit: Inherit via back propagation  RndMeth=Zero  SaturateOnIntegerOverflow=on
      settings: AttributesFormatString="LU method : %<interpMethod>\\nExtrapolation Method : %<extrapMethod>\\nBkPX = %<bp1>\\nBkPY =  %<bp2>\\nMAP  = %<tableData>"
  Interp2D : Outport
  wires:
  Lookup Table (2D)/1 -> Interp2D/1
  VarX/1 -> Lookup Table (2D)/1
  VarY/1 -> Lookup Table (2D)/2

== system AEMS_Standard_Library/LOOKUP_TABLES/AEMS_PRE_INTERP ==
  Var : Inport
  Bus Creator : BusCreator  Inputs=2  NonVirtualBus=on
      settings: AttributesFormatString=%<OutDataTypeStr>
  Prelookup : PreLookup  BreakpointsData=Cxb  IndexSearchMethod=Linear search  UseLastBreakpoint=on  BreakpointDataTypeStr=Inherit: Inherit from 'Breakpoint data'  FractionDataTypeStr=single  RndMeth=Zero
  Index_Ratio : Outport
  wires:
  Prelookup/2 -> Bus Creator/2  "Ratio"
  Prelookup/1 -> Bus Creator/1  "Index"
  Var/1 -> Prelookup/1
  Bus Creator/1 -> Index_Ratio/1

== system AEMS_Standard_Library/MATH/AEMS_CLAMP ==
  MAX : Inport  Tag=AM,In,0,1,Name,C;CMP,Port,PortWidth,SampleTime;
  Input : Inport  Tag=AM,In,0,1,Name,C;CMP,Port,PortWidth,SampleTime;  Port=2
  MIN : Inport  Tag=AM,In,0,1,Name,C;CMP,Port,PortWidth,SampleTime;  Port=3
  MinMax : MinMax  Tag=AM,Std,Inputs,1;CMP,Function,Inputs;  Inputs=2  OutDataTypeStr=Inherit: Inherit via back propagation  RndMeth=Zero  SaturateOnIntegerOverflow=on  InputSameDT=on
  MinMax1 : MinMax  Tag=AM,Std,Inputs,1;CMP,Function,Inputs;  Function=max  Inputs=2  OutDataTypeStr=Inherit: Inherit via back propagation  RndMeth=Zero  SaturateOnIntegerOverflow=on  InputSameDT=on
  Output : Outport  Tag=AM,Out,1,0,Name,NC;CMP,Port,OutputWhenDisabled,InitialOutput;  InitialOutput=0
  wires:
  MinMax/1 -> MinMax1/1
  Input/1 -> MinMax/2
  MinMax1/1 -> Output/1
  MIN/1 -> MinMax1/2
  MAX/1 -> MinMax/1

== system AEMS_Standard_Library/MATH/AEMS_DIVISION_BY_ZERO ==
  den : Inport  Tag=AM,In,0,1,Name,C;CMP,Port,PortWidth,SampleTime;
  num : Inport  Tag=AM,In,0,1,Name,C;CMP,Port,PortWidth,SampleTime;  Port=2
  ans_of_0div : Inport  Tag=AM,In,0,1,Name,C;CMP,Port,PortWidth,SampleTime;  Port=3
  Divide : Product  Inputs=*/  OutDataTypeStr=Inherit: Inherit via back propagation  RndMeth=Zero
  MinMax : MinMax  Inputs=2  OutDataTypeStr=Inherit: Inherit via back propagation  RndMeth=Zero  InputSameDT=on
  MinMax1 : MinMax  Function=max  Inputs=2  OutDataTypeStr=Inherit: Inherit via back propagation  RndMeth=Zero  InputSameDT=on
  RelationalOperator : RelationalOperator  Tag=AM,Std,2,1;CMP,Operator;  Operator=~=  OutDataTypeStr=boolean  RndMeth=Nearest  InputSameDT=on
  RelationalOperator1 : RelationalOperator  Tag=AM,Std,2,1;CMP,Operator;  Operator=>  OutDataTypeStr=boolean  RndMeth=Nearest  InputSameDT=on
  Switch1 : Switch  Tag=GEN,Threshold;AM,Switch,2,1;CMP,Threshold;  Criteria=u2 ~= 0  RndMeth=Zero  SaturateOnIntegerOverflow=on  InputSameDT=on
      settings: AttributesFormatString=Criteria=%<Criteria>
  Switch3 : Switch  Tag=GEN,Threshold;AM,Switch,2,1;CMP,Threshold;  Criteria=u2 ~= 0  RndMeth=Zero  SaturateOnIntegerOverflow=on  InputSameDT=on
      settings: AttributesFormatString=Criteria=%<Criteria>
  imm_zero : Constant  Tag=AM,Constant,0,1,Value;CMP,Value;  Value=0  OutDataTypeStr=Inherit: Inherit via back propagation
  imm_zero2 : Constant  Tag=AM,Constant,0,1,Value;CMP,Value;  Value=0  OutDataTypeStr=Inherit: Inherit via back propagation
  imm_zero3 : Constant  Tag=AM,Constant,0,1,Value;CMP,Value;  Value=Tolerence  OutDataTypeStr=Inherit: Inherit via back propagation
  imm_zero4 : Constant  Tag=AM,Constant,0,1,Value;CMP,Value;  Value=-Tolerence  OutDataTypeStr=Inherit: Inherit via back propagation
  ans : Outport  Tag=AM,Out,1,0,Name,NC;CMP,Port,OutputWhenDisabled,InitialOutput;
  wires:
  RelationalOperator/1 -> Switch1/2
  imm_zero/1 -> RelationalOperator/2
  Switch1/1 -> ans/1
  num/1 -> Divide/1
  Divide/1 -> Switch1/1
  ans_of_0div/1 -> Switch1/3
  RelationalOperator1/1 -> Switch3/2
  den/1 -> RelationalOperator/1, MinMax/1, RelationalOperator1/1, MinMax1/1
  Switch3/1 -> Divide/2
  imm_zero3/1 -> MinMax1/2
  imm_zero4/1 -> MinMax/2
  MinMax/1 -> Switch3/3
  imm_zero2/1 -> RelationalOperator1/2
  MinMax1/1 -> Switch3/1

== system AEMS_Standard_Library/MATH/AEMS_EXTRACT_INDEX ==
  X : Inport
  Vector : Inport  Port=2
  Add1 : Sum  OutDataTypeStr=Inherit: Inherit via back propagation  RndMeth=Zero  SaturateOnIntegerOverflow=on  InputSameDT=on
      settings: AttributesFormatString=SAT = %<SaturateOnIntegerOverflow>
  Constant2 : Constant  OutDataTypeStr=Inherit: Inherit via back propagation
  Constant3 : Constant  OutDataTypeStr=Inherit: Inherit via back propagation
  DataTypeConversion : DataTypeConversion  OutDataTypeStr=uint8  SaturateOnIntegerOverflow=on  RndMeth=Zero
  Data_Type_Conversion : DataTypeConversion  OutDataTypeStr=uint8  RndMeth=Zero
  IndexVector : MultiPortSwitch  Inputs=1  RndMeth=Zero  InputSameDT=on
      settings: AttributesFormatString=PortOrder=%<DataPortOrder>
  IndexVector1 : MultiPortSwitch  Inputs=1  RndMeth=Zero  InputSameDT=on
      settings: AttributesFormatString=PortOrder=%<DataPortOrder>
  MinMax : MinMax  Inputs=2  OutDataTypeStr=Inherit: Inherit via back propagation  RndMeth=Zero  InputSameDT=on
  MinMax1 : MinMax  Function=max  Inputs=2  OutDataTypeStr=Inherit: Inherit via back propagation  RndMeth=Zero  InputSameDT=on
  RelationalOperator8 : RelationalOperator  OutDataTypeStr=boolean  RndMeth=Nearest  InputSameDT=on
  Relational_Operator : RelationalOperator  Operator===  OutDataTypeStr=boolean  RndMeth=Nearest  InputSameDT=on
  Sum_of_Elements : Sum  Inputs=+  OutDataTypeStr=Inherit: Inherit via back propagation  RndMeth=Zero  SaturateOnIntegerOverflow=on  InputSameDT=on
      settings: AttributesFormatString=SAT = %<SaturateOnIntegerOverflow>
  SumofElements : Sum  Inputs=+  OutDataTypeStr=Inherit: Inherit via back propagation  RndMeth=Zero  SaturateOnIntegerOverflow=on  InputSameDT=on
      settings: AttributesFormatString=SAT = %<SaturateOnIntegerOverflow>
  Index_prev : Outport
  Index_nxt : Outport  Port=2
  Next_Value : Outport  Port=3
  Previous_Value : Outport  Port=4
  wires:
  Sum_of_Elements/1 -> MinMax/2
  Relational_Operator/1 -> Data_Type_Conversion/1
  Data_Type_Conversion/1 -> Sum_of_Elements/1
  IndexVector1/1 -> Previous_Value/1
  IndexVector/1 -> Next_Value/1
  Vector/1 -> RelationalOperator8/2, Relational_Operator/2, Relational_Operator/1, IndexVector/2, IndexVector1/2
  Add1/1 -> MinMax/1
  MinMax/1 -> IndexVector/1, Index_nxt/1
  X/1 -> RelationalOperator8/1
  Constant3/1 -> Add1/2
  Constant2/1 -> MinMax1/1
  SumofElements/1 -> MinMax1/2
  MinMax1/1 -> Add1/1, IndexVector1/1, Index_prev/1
  DataTypeConversion/1 -> SumofElements/1
  RelationalOperator8/1 -> DataTypeConversion/1

== system AEMS_Standard_Library/MATH/AEMS_IGN_TO_PHY ==
  Order_vector : Inport
  Replace : Inport  Port=2
  In : Inport  Port=3
  Constant1 : Constant  Value=nb_cyl_max  OutDataTypeStr=Inherit: Inherit via back propagation
  Constant2 : Constant  Value=[1:nb_cyl_max]  OutDataTypeStr=uint8
  Constant3 : Constant  OutDataTypeStr=Inherit: Inherit via back propagation
  Constant4 : Constant  Value=false
  Constant6 : Constant  Value=0  OutDataTypeStr=Inherit: Inherit via back propagation
  Inverse_order : Subsystem
  MinMax : MinMax  Function=max  Inputs=2  OutDataTypeStr=Inherit: Inherit via back propagation  RndMeth=Zero  InputSameDT=on
  MinMax1 : MinMax  Inputs=2  OutDataTypeStr=Inherit: Inherit via back propagation  RndMeth=Zero  InputSameDT=on
  RelationalOperator1 : RelationalOperator  Operator===  OutDataTypeStr=boolean  RndMeth=Nearest  InputSameDT=on
  Selector : Selector  InputPortWidth=nb_cyl_max  IndexOptions=Index vector (port)  Indices=[1 3]  OutputSizes=1
      settings: AttributesFormatString=Index mode: %<IndexMode>\nInput Port Width : %<InputPortWidth>
  Selector2 : Selector  InputPortWidth=6  IndexOptions=Index vector (port)  Indices=[1 3]  OutputSizes=1
      settings: AttributesFormatString=Index mode: %<IndexMode>\nInput Port Width: %<InputPortWidth>
  Switch : Switch  Criteria=u2 ~= 0  RndMeth=Zero  SaturateOnIntegerOverflow=on  InputSameDT=on
      settings: AttributesFormatString=Criteria=%<Criteria>
  UnitDelay : UnitDelay  InitialCondition=true  SampleTime=-1
      settings: AttributesFormatString=IC = %<X0>
  Out : Outport
  wires:
  UnitDelay/1 -> Inverse_order/Enable
  Constant4/1 -> UnitDelay/1
  Constant6/1 -> RelationalOperator1/1
  RelationalOperator1/1 -> Switch/2
  Replace/1 -> Switch/1
  Constant3/1 -> MinMax/2
  MinMax/1 -> Selector/2
  Selector/1 -> Switch/3
  Switch/1 -> Out/1
  In/1 -> Selector/1
  Constant2/1 -> Selector2/2
  Order_vector/1 -> Inverse_order/1(Order_vector)
  Selector2/1 -> RelationalOperator1/2, MinMax/1
  Constant1/1 -> MinMax1/1
  Inverse_order/1(Inverted_vector) -> MinMax1/2
  MinMax1/1 -> Selector2/1

== system AEMS_Standard_Library/MATH/AEMS_MATRIX_INVERSION ==
  Matrix_Input : Inport
  Alternate_Input : Inport  Port=2
  Co-factors of the Matrix : Subsystem
  Determinant of the Matrix : Subsystem
  Elements of the Matrix : Subsystem
  If : If  IfExpression=u1 ~= 0
  Matrix_inversion : Subsystem  TreatAsAtomicUnit=on
  Matrix_inversion_not_possible : Subsystem  TreatAsAtomicUnit=on
  Merge : Merge  InitialOutput=0
      settings: AttributesFormatString=<initial=%<InitialOutput>>
  Inverted_Matrix : Outport
  wires:
  Elements of the Matrix/5(m11) -> Determinant of the Matrix/5(m11), Co-factors of the Matrix/5(m11)
  Elements of the Matrix/2(m01) -> Determinant of the Matrix/2(m01), Co-factors of the Matrix/2(m01)
  Determinant of the Matrix/3(Co_m12) -> Co-factors of the Matrix/11(Co_m10)
  Elements of the Matrix/7(m20) -> Determinant of the Matrix/7(m20), Co-factors of the Matrix/7(m21)
  Elements of the Matrix/3(m02) -> Determinant of the Matrix/3(m02), Co-factors of the Matrix/3(m02)
  Elements of the Matrix/4(m10) -> Determinant of the Matrix/4(m10), Co-factors of the Matrix/4(m10)
  Determinant of the Matrix/2(Co_m11) -> Co-factors of the Matrix/10(Co_m00)
  Co-factors of the Matrix/1(Adj_m) -> Matrix_inversion/1(Adj_m)
  Elements of the Matrix/9(m22) -> Determinant of the Matrix/9(m22), Co-factors of the Matrix/9(m23)
  Elements of the Matrix/6(m12) -> Determinant of the Matrix/6(m12), Co-factors of the Matrix/6(m12)
  Determinant of the Matrix/4(Co_m13) -> Co-factors of the Matrix/12(Co_m20)
  Elements of the Matrix/1(m00) -> Determinant of the Matrix/1(m00), Co-factors of the Matrix/1(m00)
  Elements of the Matrix/8(m21) -> Determinant of the Matrix/8(m21), Co-factors of the Matrix/8(m22)
  Matrix_Input/1 -> Elements of the Matrix/1(m_3x3)
  Determinant of the Matrix/1(Det_m) -> Matrix_inversion/2(Det_m), If/1
  Merge/1 -> Inverted_Matrix/1
  If/1 -> Matrix_inversion/Action
  If/2 -> Matrix_inversion_not_possible/Action
  Matrix_inversion/1(" Inverted_Matrix") -> Merge/1
  Matrix_inversion_not_possible/1(" Alternate_Output") -> Merge/2
  Alternate_Input/1 -> Matrix_inversion/3(Alternate_Input), Matrix_inversion_not_possible/1(Alternate_Input)

== system AEMS_Standard_Library/MATH/AEMS_PHY_TO_IGN ==
  Order_vector : Inport
  Replace : Inport  Port=2
  In : Inport  Port=3
  Constant1 : Constant  Value=nb_cyl_max  OutDataTypeStr=Inherit: Inherit via back propagation
  Constant2 : Constant  Value=[1:nb_cyl_max]  OutDataTypeStr=uint8
  Constant3 : Constant  OutDataTypeStr=Inherit: Inherit via back propagation
  Constant6 : Constant  Value=0  OutDataTypeStr=Inherit: Inherit via back propagation
  MinMax : MinMax  Function=max  Inputs=2  OutDataTypeStr=Inherit: Inherit via back propagation  RndMeth=Zero  InputSameDT=on
  MinMax1 : MinMax  Inputs=2  OutDataTypeStr=Inherit: Inherit via back propagation  RndMeth=Zero  InputSameDT=on
  RelationalOperator1 : RelationalOperator  Operator===  OutDataTypeStr=boolean  RndMeth=Nearest  InputSameDT=on
  Selector : Selector  InputPortWidth=nb_cyl_max  IndexOptions=Index vector (port)  Indices=[1 3]  OutputSizes=1
      settings: AttributesFormatString=Index mode: %<IndexMode>\nInput Port Width : %<InputPortWidth>
  Selector2 : Selector  InputPortWidth=6  IndexOptions=Index vector (port)  Indices=[1 3]  OutputSizes=1
      settings: AttributesFormatString=Index mode: %<IndexMode>\nInput Port Width: %<InputPortWidth>
  Switch : Switch  Criteria=u2 ~= 0  RndMeth=Zero  SaturateOnIntegerOverflow=on  InputSameDT=on
      settings: AttributesFormatString=Criteria=%<Criteria>
  Out : Outport
  wires:
  Constant6/1 -> RelationalOperator1/1
  RelationalOperator1/1 -> Switch/2
  Replace/1 -> Switch/1
  Constant3/1 -> MinMax/2
  MinMax/1 -> Selector/2
  Selector/1 -> Switch/3
  Switch/1 -> Out/1
  In/1 -> Selector/1
  Constant2/1 -> Selector2/2
  Selector2/1 -> RelationalOperator1/2, MinMax/1
  Constant1/1 -> MinMax1/1
  Order_vector/1 -> MinMax1/2
  MinMax1/1 -> Selector2/1

== system AEMS_Standard_Library/MATH/AEMS_PROTECTED_DIVISION ==
  num : Inport
  den : Inport  Port=2
  Abs : Abs  RndMeth=Zero
      settings: AttributesFormatString=SAT = %<SaturateOnIntegerOverflow>
  Den_Tol : Constant  Value=tolerance  OutDataTypeStr=Inherit: Inherit via back propagation
  Divide : Product  Inputs=*/  OutDataTypeStr=Inherit: Inherit via back propagation  RndMeth=Zero
  RelationalOperator : RelationalOperator  Operator=>  OutDataTypeStr=boolean  RndMeth=Zero  InputSameDT=on
  Switch : Switch  Criteria=u2 ~= 0  RndMeth=Zero
      settings: AttributesFormatString=Criteria=%<Criteria>
  result : Outport
  wires:
  Abs/1 -> RelationalOperator/1
  Den_Tol/1 -> Switch/3, RelationalOperator/2
  den/1 -> Switch/1, Abs/1
  RelationalOperator/1 -> Switch/2
  num/1 -> Divide/1
  Switch/1 -> Divide/2
  Divide/1 -> result/1

== system AEMS_Standard_Library/MATH/AEMS_SORT ==
  Vector_to_sort : Inport
  Index : Inport  Port=2
  AEMS_SORT_MEDIAN : AEMS_Standard_Library/SUB/AEMS_SORT_MEDIAN  Tag=[LIB]
      settings: AttributesFormatString=%<MaskType>
  For_loop_1 : Subsystem  TreatAsAtomicUnit=on
  Sorted_vector 0:N : Outport
  Median_Out : Outport  Port=2
  wires:
  AEMS_SORT_MEDIAN/1 -> Median_Out/1
  Index/1 -> AEMS_SORT_MEDIAN/2, For_loop_1/2(Selected_index)
  For_loop_1/1(Sorted_vector) -> AEMS_SORT_MEDIAN/1, Sorted_vector 0:N/1
  Vector_to_sort/1 -> For_loop_1/1(Vector_to_sort)

== system AEMS_Standard_Library/MATH/AEMS_SQRT ==
  note: It can perform square root operation for both signed and unsigned values or
      |  it can perform reciprocal square root operation.
  Input : Inport
  Sqrt : Sqrt  Operator=signedSqrt  RndMeth=Zero  SaturateOnIntegerOverflow=on
  Output : Outport
  wires:
  Input/1 -> Sqrt/1
  Sqrt/1 -> Output/1

== system AEMS_Standard_Library/MEM/AEMS_NVM_WRITEONFLY ==
  In1 : Inport
  PortType : TriggerPort  VariantControl=Variant  PortDimensions=1
      settings: AttributesFormatString=StatesWhenEnabling = %<StatesWhenEnabling>
  Terminator1 : Terminator
  wires:
  In1/1 -> Terminator1/1

== system AEMS_Standard_Library/MEM/AEMS_NVM_WRITEONFLY_ENABLE ==
  Enable : EnablePort
      settings: AttributesFormatString=StatesWhenEnabling = %<StatesWhenEnabling>

== system AEMS_Standard_Library/SAFETY/AEMS_SAFETY_AND_REGULATION ==
